simulink model "gm_wlanhdlTimeAndFrequencySynchronization"  (R2025a)
settings: Solver=FixedStepDiscrete  StartTime=0.0  StopTime=stopTime  RelTol=1e-3
InitFcn:
  | wlanFrontEndInit;
undefined symbols (not defined in the file or in its folder): a, b, c, Hd, wlanConfig
libraries: simulink x95, hdlsllib x16, hdlmdlgenlib x12, dspsrcs4 x3, dspsigops x3, dsphdlsigops2 x2, dsphdlfiltering2 x2
(part 7 of 11)

== system gm_wlanhdlTimeAndFrequencySynchronization/WLANTimeAndFrequencySynchronization/Coarse CFO Estimation and Correction/Coarse CFO Estimation/Iteration8 ==
  xin : Inport  OutDataTypeStr=fixdt(1, 32, 19)  SampleTime=6.25e-09
  yin : Inport  Port=2  OutDataTypeStr=fixdt(1, 32, 19)  SampleTime=6.25e-09
  zin : Inport  Port=3  OutDataTypeStr=fixdt(1, 34, 33)  SampleTime=6.25e-09
  lut_value : Inport  Port=4  OutDataTypeStr=fixdt(0, 31, 33)  SampleTime=6.25e-09
  idx : Inport  Port=5  OutDataTypeStr=fixdt(0, 6, 0)  SampleTime=6.25e-09
  MuxX : Switch  Criteria=u2 ~= 0  Threshold="fi(0,0,1,0,\"hex\",\"0\")"  OutDataTypeStr=fixdt(1, 32, 19)  SampleTime=6.25e-09  SaturateOnIntegerOverflow=off  InputSameDT=off
  MuxY : Switch  Criteria=u2 ~= 0  Threshold="fi(0,0,1,0,\"hex\",\"0\")"  OutDataTypeStr=fixdt(1, 32, 19)  SampleTime=6.25e-09  SaturateOnIntegerOverflow=off  InputSameDT=off
  MuxZ : Switch  Criteria=u2 ~= 0  Threshold="fi(0,0,1,0,\"hex\",\"0\")"  OutDataTypeStr=fixdt(1, 34, 33)  SampleTime=6.25e-09  SaturateOnIntegerOverflow=off  InputSameDT=off
  XAdder : Sum  OutDataTypeStr=fixdt(1, 32, 19)  SampleTime=6.25e-09
  XSubtractor : Sum  Inputs=+-  OutDataTypeStr=fixdt(1, 32, 19)  AccumDataTypeStr=fixdt(1, 32, 19)  SampleTime=6.25e-09
  YAdder : Sum  OutDataTypeStr=fixdt(1, 32, 19)  SampleTime=6.25e-09
  YSub : Sum  Inputs=+-  OutDataTypeStr=fixdt(1, 32, 19)  AccumDataTypeStr=fixdt(1, 32, 19)  SampleTime=6.25e-09
  ZAdder : Sum  OutDataTypeStr=fixdt(1, 34, 33)  SampleTime=6.25e-09
  ZSub : Sum  Inputs=+-  OutDataTypeStr=fixdt(1, 34, 33)  AccumDataTypeStr=fixdt(1, 34, 33)  SampleTime=6.25e-09
  compare : simulink/Logic and Bit Operations/Compare To Constant  relop=<  const=double(0)  OutDataTypeStr=boolean
  dynamic_shift : ArithShift  BitShiftNumberSource=Input port  BitShiftDirection=Right
      settings: InputPortMap=u0,p1
  dynamic_shift1 : ArithShift  BitShiftNumberSource=Input port  BitShiftDirection=Right
      settings: InputPortMap=u0,p1
  rd_{0..9} (10 alike) : Delay  DelayLength=double(1)  InitialCondition=0  SampleTime=6.25e-09
  xout : Outport  OutDataTypeStr=fixdt(1, 32, 19)  SampleTime=6.25e-09
  yout : Outport  Port=2  OutDataTypeStr=fixdt(1, 32, 19)  SampleTime=6.25e-09
  zout : Outport  Port=3  OutDataTypeStr=fixdt(1, 34, 33)  SampleTime=6.25e-09
  wires:
  MuxY/1 -> yout/1
  rd_4/1 -> MuxX/3
  rd_3/1 -> MuxX/2, MuxY/2, MuxZ/2
  rd_2/1 -> MuxX/1
  rd_6/1 -> MuxY/3
  rd_5/1 -> MuxY/1
  XAdder/1 -> rd_4/1
  XSubtractor/1 -> rd_2/1
  ZAdder/1 -> rd_9/1
  MuxX/1 -> xout/1
  rd_8/1 -> MuxZ/1
  ZSub/1 -> rd_8/1
  yin/1 -> rd_1/1
  xin/1 -> rd_0/1
  idx/1 -> dynamic_shift1/2, dynamic_shift/2
  rd_1/1 -> compare/1, YAdder/1, dynamic_shift1/1, YSub/1
  zin/1 -> rd_7/1
  YSub/1 -> rd_6/1
  rd_0/1 -> dynamic_shift/1, XSubtractor/1, XAdder/1
  MuxZ/1 -> zout/1
  dynamic_shift/1 -> YSub/2, YAdder/2
  YAdder/1 -> rd_5/1
  rd_9/1 -> MuxZ/3
  rd_7/1 -> ZSub/1, ZAdder/1
  compare/1 -> rd_3/1
  lut_value/1 -> ZAdder/2, ZSub/2
  dynamic_shift1/1 -> XAdder/2, XSubtractor/2

== system gm_wlanhdlTimeAndFrequencySynchronization/WLANTimeAndFrequencySynchronization/Coarse CFO Estimation and Correction/Coarse CFO Estimation/Iteration9 ==
  xin : Inport  OutDataTypeStr=fixdt(1, 32, 19)  SampleTime=6.25e-09
  yin : Inport  Port=2  OutDataTypeStr=fixdt(1, 32, 19)  SampleTime=6.25e-09
  zin : Inport  Port=3  OutDataTypeStr=fixdt(1, 34, 33)  SampleTime=6.25e-09
  lut_value : Inport  Port=4  OutDataTypeStr=fixdt(0, 31, 33)  SampleTime=6.25e-09
  idx : Inport  Port=5  OutDataTypeStr=fixdt(0, 6, 0)  SampleTime=6.25e-09
  MuxX : Switch  Criteria=u2 ~= 0  Threshold="fi(0,0,1,0,\"hex\",\"0\")"  OutDataTypeStr=fixdt(1, 32, 19)  SampleTime=6.25e-09  SaturateOnIntegerOverflow=off  InputSameDT=off
  MuxY : Switch  Criteria=u2 ~= 0  Threshold="fi(0,0,1,0,\"hex\",\"0\")"  OutDataTypeStr=fixdt(1, 32, 19)  SampleTime=6.25e-09  SaturateOnIntegerOverflow=off  InputSameDT=off
  MuxZ : Switch  Criteria=u2 ~= 0  Threshold="fi(0,0,1,0,\"hex\",\"0\")"  OutDataTypeStr=fixdt(1, 34, 33)  SampleTime=6.25e-09  SaturateOnIntegerOverflow=off  InputSameDT=off
  XAdder : Sum  OutDataTypeStr=fixdt(1, 32, 19)  SampleTime=6.25e-09
  XSubtractor : Sum  Inputs=+-  OutDataTypeStr=fixdt(1, 32, 19)  AccumDataTypeStr=fixdt(1, 32, 19)  SampleTime=6.25e-09
  YAdder : Sum  OutDataTypeStr=fixdt(1, 32, 19)  SampleTime=6.25e-09
  YSub : Sum  Inputs=+-  OutDataTypeStr=fixdt(1, 32, 19)  AccumDataTypeStr=fixdt(1, 32, 19)  SampleTime=6.25e-09
  ZAdder : Sum  OutDataTypeStr=fixdt(1, 34, 33)  SampleTime=6.25e-09
  ZSub : Sum  Inputs=+-  OutDataTypeStr=fixdt(1, 34, 33)  AccumDataTypeStr=fixdt(1, 34, 33)  SampleTime=6.25e-09
  compare : simulink/Logic and Bit Operations/Compare To Constant  relop=<  const=double(0)  OutDataTypeStr=boolean
  dynamic_shift : ArithShift  BitShiftNumberSource=Input port  BitShiftDirection=Right
      settings: InputPortMap=u0,p1
  dynamic_shift1 : ArithShift  BitShiftNumberSource=Input port  BitShiftDirection=Right
      settings: InputPortMap=u0,p1
  rd_{0..9} (10 alike) : Delay  DelayLength=double(1)  InitialCondition=0  SampleTime=6.25e-09
  xout : Outport  OutDataTypeStr=fixdt(1, 32, 19)  SampleTime=6.25e-09
  yout : Outport  Port=2  OutDataTypeStr=fixdt(1, 32, 19)  SampleTime=6.25e-09
  zout : Outport  Port=3  OutDataTypeStr=fixdt(1, 34, 33)  SampleTime=6.25e-09
  wires:
  MuxZ/1 -> zout/1
  rd_4/1 -> MuxX/3
  rd_2/1 -> MuxX/1
  MuxY/1 -> yout/1
  XAdder/1 -> rd_4/1
  XSubtractor/1 -> rd_2/1
  YAdder/1 -> rd_5/1
  yin/1 -> rd_1/1
  YSub/1 -> rd_6/1
  lut_value/1 -> ZSub/2, ZAdder/2
  rd_3/1 -> MuxX/2, MuxZ/2, MuxY/2
  compare/1 -> rd_3/1
  dynamic_shift/1 -> YAdder/2, YSub/2
  rd_5/1 -> MuxY/1
  xin/1 -> rd_0/1
  MuxX/1 -> xout/1
  zin/1 -> rd_7/1
  rd_6/1 -> MuxY/3
  rd_0/1 -> dynamic_shift/1, XSubtractor/1, XAdder/1
  idx/1 -> dynamic_shift/2, dynamic_shift1/2
  rd_8/1 -> MuxZ/1
  rd_7/1 -> ZSub/1, ZAdder/1
  rd_9/1 -> MuxZ/3
  dynamic_shift1/1 -> XSubtractor/2, XAdder/2
  ZSub/1 -> rd_8/1
  rd_1/1 -> compare/1, dynamic_shift1/1, YAdder/1, YSub/1
  ZAdder/1 -> rd_9/1

== system gm_wlanhdlTimeAndFrequencySynchronization/WLANTimeAndFrequencySynchronization/Coarse CFO Estimation and Correction/Coarse CFO Estimation/QuadrantCorrection ==
  zin : Inport  OutDataTypeStr=fixdt(1, 34, 33)  SampleTime=6.25e-09
  QA_Control : Inport  Port=2  OutDataTypeStr=fixdt(0, 5, 0)  SampleTime=6.25e-09
  Negation : Gain  Gain="fi(0,1,2,0,\"hex\",\"3\")"  ParamDataTypeStr=fixdt(1, 2, 0)  OutDataTypeStr=fixdt(1, 34, 33)  SampleTime=6.25e-09
  adder : Sum  OutDataTypeStr=fixdt(1, 34, 33)  SampleTime=6.25e-09
  dtc : hdlmdlgenlib/Buffer
  extract : simulink/Logic and Bit Operations/Extract Bits  bitsToExtract=Range of bits  numBits=8  bitIdxRange=[2 2]  outScalingMode=Treat bit field as an integer
  extract1 : simulink/Logic and Bit Operations/Extract Bits  bitsToExtract=Range of bits  numBits=8  bitIdxRange=[0 1]  outScalingMode=Treat bit field as an integer
  mux : MultiPortSwitch  DataPortOrder=Zero-based contiguous  Inputs=2  DiagnosticForDefault=None  zeroidx=on  OutDataTypeStr=fixdt(1, 34, 33)  SampleTime=6.25e-09  SaturateOnIntegerOverflow=off  InputSameDT=off
  mux1 : MultiPortSwitch  DataPortOrder=Zero-based contiguous  Inputs=4  DiagnosticForDefault=None  zeroidx=on  OutDataTypeStr=fixdt(1, 34, 33)  SampleTime=6.25e-09  SaturateOnIntegerOverflow=off  InputSameDT=off
  mux2 : MultiPortSwitch  DataPortOrder=Zero-based contiguous  Inputs=2  DiagnosticForDefault=None  zeroidx=on  OutDataTypeStr=fixdt(1, 34, 33)  SampleTime=6.25e-09  SaturateOnIntegerOverflow=off  InputSameDT=off
  mux3 : MultiPortSwitch  DataPortOrder=Zero-based contiguous  Inputs=2  DiagnosticForDefault=None  zeroidx=on  OutDataTypeStr=fixdt(1, 34, 33)  SampleTime=6.25e-09  SaturateOnIntegerOverflow=off  InputSameDT=off
  mux6out_wire : hdlmdlgenlib/Buffer
  pidivtwoconstant : Constant  Value=0.5  OutDataTypeStr=fixdt(1, 34, 33)  SampleTime=6.25e-09
  pidivtwoconstant1 : Constant  Value=0.999999999883584678173065185546875  OutDataTypeStr=fixdt(1, 34, 33)  SampleTime=6.25e-09
  pidivtwoconstant2 : Constant  Value=-1  OutDataTypeStr=fixdt(1, 34, 33)  SampleTime=6.25e-09
  pidivtwoconstant3 : Constant  Value=0  OutDataTypeStr=fixdt(1, 34, 33)  SampleTime=6.25e-09
  pidivtwosub : Sum  Inputs=+-  OutDataTypeStr=fixdt(1, 34, 33)  AccumDataTypeStr=fixdt(1, 34, 33)  SampleTime=6.25e-09
  rd_{0,2..3,6..7} (5 alike) : Delay  DelayLength=double(1)  InitialCondition=0  SampleTime=6.25e-09
  rd_{1,4..5,8..9} (5 alike) : Delay  DelayLength=double(2)  InitialCondition=0  SampleTime=6.25e-09
  slice : hdlsllib/Logic and Bit Operations/Bit Slice  lidx=double(3)  ridx=double(3)
  slice1 : hdlsllib/Logic and Bit Operations/Bit Slice  lidx=double(4)  ridx=double(4)
  subfmux : Sum  Inputs=+-  OutDataTypeStr=fixdt(1, 34, 33)  AccumDataTypeStr=fixdt(1, 34, 33)  SampleTime=6.25e-09
  zout : Outport  OutDataTypeStr=fixdt(1, 34, 33)  SampleTime=6.25e-09
  wires:
  mux6out_wire/1 -> zout/1
  pidivtwoconstant2/1 -> adder/1
  slice1/1 -> rd_1/1
  slice/1 -> rd_4/1
  pidivtwoconstant/1 -> pidivtwosub/1
  rd_0/1 -> extract/1, slice/1, slice1/1, extract1/1
  pidivtwosub/1 -> mux/2
  rd_3/1 -> rd_6/1, Negation/1
  dtc/1 -> pidivtwosub/2, mux/3
  extract/1 -> mux/1
  QA_Control/1 -> rd_0/1
  adder/1 -> rd_9/1
  Negation/1 -> rd_7/1
  extract1/1 -> rd_5/1
  rd_2/1 -> dtc/1
  mux3/1 -> mux6out_wire/1
  pidivtwoconstant1/1 -> subfmux/1, mux2/3
  rd_6/1 -> mux1/2
  rd_5/1 -> mux1/1
  subfmux/1 -> rd_8/1
  rd_7/1 -> mux1/3
  rd_8/1 -> mux1/4
  rd_9/1 -> mux1/5
  rd_1/1 -> mux3/1
  rd_4/1 -> mux2/1
  mux1/1 -> mux2/2
  mux/1 -> rd_3/1, adder/2, subfmux/2
  zin/1 -> rd_2/1
  mux2/1 -> mux3/2
  pidivtwoconstant3/1 -> mux3/3

== system gm_wlanhdlTimeAndFrequencySynchronization/WLANTimeAndFrequencySynchronization/Coarse CFO Estimation and Correction/Coarse CFO Estimation/QuadrantMapper ==
  xin : Inport  OutDataTypeStr=fixdt(1, 32, 19)  SampleTime=5e-08
  yin : Inport  Port=2  OutDataTypeStr=fixdt(1, 32, 19)  SampleTime=5e-08
  Delayin1 : UnitDelay  InitialCondition=double(0)  SampleTime=5e-08
  Delayin11 : RateTransition  InitialCondition=double(0)  OutPortSampleTimeOpt=Multiple of input port sample time  OutPortSampleTimeMultiple=8
  Delayin2 : UnitDelay  InitialCondition=double(0)  SampleTime=5e-08
  Delayin21 : RateTransition  InitialCondition=double(0)  OutPortSampleTimeOpt=Multiple of input port sample time  OutPortSampleTimeMultiple=8
  DelayxAbs : RateTransition  InitialCondition=double(0)  OutPortSampleTimeOpt=Multiple of input port sample time  OutPortSampleTimeMultiple=8
  DelayxAbs_absorbed : Delay  DelayLength=0
  DelayyAbs : RateTransition  InitialCondition=double(0)  OutPortSampleTimeOpt=Multiple of input port sample time  OutPortSampleTimeMultiple=8
  DelayyAbs_absorbed : Delay  DelayLength=0
  abs : Abs  SampleTime=6.25e-09  OutDataTypeStr=fixdt(1, 32, 19)  SaturateOnIntegerOverflow=off
  abs1 : Abs  SampleTime=6.25e-09  OutDataTypeStr=fixdt(1, 32, 19)  SaturateOnIntegerOverflow=off
  and : Logic  AllPortsSameDT=off  OutDataTypeStr=fixdt(0, 1, 0)  SampleTime=6.25e-09
  and1 : Logic  AllPortsSameDT=off  OutDataTypeStr=fixdt(0, 1, 0)  SampleTime=6.25e-09
  compare : simulink/Logic and Bit Operations/Compare To Constant  relop=<  const=double(0)  OutDataTypeStr=boolean
  compare1 : simulink/Logic and Bit Operations/Compare To Constant  relop===  const=double(0)  OutDataTypeStr=boolean
  compare2 : simulink/Logic and Bit Operations/Compare To Constant  relop=>=  const=double(0)  OutDataTypeStr=boolean
  compare3 : simulink/Logic and Bit Operations/Compare To Constant  relop=<  const=double(0)  OutDataTypeStr=boolean
  concatQCControl : hdlsllib/Logic and Bit Operations/Bit Concat  numInputs=5
  crp_out_delay : Delay  DelayLength=double(1)  InitialCondition=0  SampleTime=6.25e-09
  crp_out_delay1 : Delay  DelayLength=double(1)  InitialCondition=0  SampleTime=6.25e-09
  dtc : hdlmdlgenlib/Buffer
  dtc1 : hdlmdlgenlib/Buffer
  in0_repeat : RateTransition  Integrity=off  Deterministic=off  OutPortSampleTimeOpt=Multiple of input port sample time  OutPortSampleTimeMultiple=1/8
  in0_repeat1 : RateTransition  Integrity=off  Deterministic=off  OutPortSampleTimeOpt=Multiple of input port sample time  OutPortSampleTimeMultiple=1/8
  in1_repeat : RateTransition  Integrity=off  Deterministic=off  OutPortSampleTimeOpt=Multiple of input port sample time  OutPortSampleTimeMultiple=1/8
  in1_repeat1 : RateTransition  Integrity=off  Deterministic=off  OutPortSampleTimeOpt=Multiple of input port sample time  OutPortSampleTimeMultiple=1/8
  in2_repeat : RateTransition  Integrity=off  Deterministic=off  OutPortSampleTimeOpt=Multiple of input port sample time  OutPortSampleTimeMultiple=1/8
  in3_repeat : RateTransition  Integrity=off  Deterministic=off  OutPortSampleTimeOpt=Multiple of input port sample time  OutPortSampleTimeMultiple=1/8
  mux : MultiPortSwitch  DataPortOrder=Zero-based contiguous  Inputs=2  DiagnosticForDefault=None  zeroidx=on  OutDataTypeStr=fixdt(1, 32, 19)  SampleTime=6.25e-09  SaturateOnIntegerOverflow=off  InputSameDT=off
  mux1 : MultiPortSwitch  DataPortOrder=Zero-based contiguous  Inputs=2  DiagnosticForDefault=None  zeroidx=on  OutDataTypeStr=fixdt(1, 32, 19)  SampleTime=6.25e-09  SaturateOnIntegerOverflow=off  InputSameDT=off
  qcControl_wire : hdlmdlgenlib/Buffer
  rd_{0..10,41} (12 alike) : Delay  DelayLength=double(1)  InitialCondition=0  SampleTime=6.25e-09
  rd_01 : Delay  DelayLength=double(1)  InitialCondition=0  SampleTime=6.25e-09
  relop : RelationalOperator  Operator=>  OutDataTypeStr=fixdt(0, 1, 0)  SampleTime=6.25e-09
  xout : Outport  OutDataTypeStr=fixdt(1, 32, 19)  SampleTime=6.25e-09
  yout : Outport  Port=2  OutDataTypeStr=fixdt(1, 32, 19)  SampleTime=6.25e-09
  QA_Control : Outport  Port=3  OutDataTypeStr=fixdt(0, 5, 0)  SampleTime=6.25e-09
  wires:
  dtc/1 -> yout/1
  qcControl_wire/1 -> QA_Control/1
  mux1/1 -> dtc1/1
  concatQCControl/1 -> qcControl_wire/1
  rd_7/1 -> concatQCControl/3, mux/1, mux1/1
  dtc1/1 -> xout/1
  and/1 -> concatQCControl/2
  and1/1 -> concatQCControl/1
  rd_8/1 -> concatQCControl/5
  rd_9/1 -> mux/2, mux1/3
  rd_4/1 -> and/2, concatQCControl/4
  rd_3/1 -> and1/2
  rd_6/1 -> relop/2, rd_10/1
  crp_out_delay/1 -> DelayyAbs/1
  rd_10/1 -> mux/3, mux1/2
  crp_out_delay1/1 -> DelayxAbs/1
  yin/1 -> in0_repeat1/1
  mux/1 -> dtc/1
  DelayyAbs_absorbed/1 -> in3_repeat/1
  abs1/1 -> crp_out_delay1/1
  compare/1 -> rd_4/1
  Delayin21/1 -> Delayin2/1
  compare2/1 -> rd_3/1
  relop/1 -> rd_7/1
  compare3/1 -> rd_8/1
  rd_2/1 -> compare/1, compare2/1
  rd_01/1 -> abs/1
  abs/1 -> crp_out_delay/1
  Delayin1/1 -> in0_repeat/1
  in1_repeat/1 -> rd_0/1
  Delayin11/1 -> Delayin1/1
  rd_41/1 -> abs1/1
  in1_repeat1/1 -> Delayin11/1, rd_41/1
  rd_5/1 -> relop/1, rd_9/1
  xin/1 -> in1_repeat1/1
  DelayxAbs/1 -> DelayxAbs_absorbed/1
  DelayyAbs/1 -> DelayyAbs_absorbed/1
  in0_repeat/1 -> rd_2/1
  DelayxAbs_absorbed/1 -> in2_repeat/1
  rd_1/1 -> and/1, and1/1
  rd_0/1 -> compare1/1, compare3/1
  in0_repeat1/1 -> rd_01/1, Delayin21/1
  in3_repeat/1 -> rd_6/1
  Delayin2/1 -> in1_repeat/1
  in2_repeat/1 -> rd_5/1
  compare1/1 -> rd_1/1

== system gm_wlanhdlTimeAndFrequencySynchronization/WLANTimeAndFrequencySynchronization/Coarse CFO Estimation and Correction/Coarse CFO Estimation/Sample FreqOff ==
  freqOffIn : Inport  OutDataTypeStr=fixdt(1, 34, 33)  PortDimensions=1  SampleTime=5e-08
  enb : Inport  Port=2  OutDataTypeStr=boolean  PortDimensions=1  SampleTime=5e-08
  rst : Inport  Port=3  OutDataTypeStr=boolean  PortDimensions=1  SampleTime=5e-08
  Sample FreqOff : MATLAB Function  TreatAsAtomicUnit=on
  freqOffOut : Outport  SampleTime=5e-08  VectorParamsAs1DForOutWhenUnconnected=off
  wires:
  Sample FreqOff/1(freqOffOut) -> freqOffOut/1
  rst/1 -> Sample FreqOff/3(rst)
  enb/1 -> Sample FreqOff/2(enb)
  freqOffIn/1 -> Sample FreqOff/1(freqOffIn)

== system gm_wlanhdlTimeAndFrequencySynchronization/WLANTimeAndFrequencySynchronization/Coarse Time Sync/Correlator/MagnitudeSquared ==
  dataIn : Inport  OutDataTypeStr=fixdt(1, 33, 26)  PortDimensions=1  SampleTime=6.25e-09
      settings: SignalType=complex
  validIn : Inport  Port=2  OutDataTypeStr=boolean  PortDimensions=1  SampleTime=6.25e-09
  Add : Sum  OutDataTypeStr=fixdt(1, 66, 52)  AccumDataTypeStr=fixdt(1, 66, 52)  SampleTime=6.25e-09
  Complex to Real-Imag : ComplexToRealImag  SampleTime=6.25e-09
  Delay{,1..3} (4 alike) : Delay  DelayLength=double(1)  InitialCondition=0  SampleTime=5e-08
  Delay{4..5,11,21,31,41,61} (7 alike) : RateTransition  InitialCondition=double(0)  OutPortSampleTimeOpt=Multiple of input port sample time  OutPortSampleTimeMultiple=8
  Delay4_absorbed : Delay  DelayLength=0
  Delay5_absorbed : Delay  DelayLength=0
  Delay6 : Delay  DelayLength=double(2)  InitialCondition=0  SampleTime=5e-08
  HwModeRegister{,1..3} (4 alike) : Delay  DelayLength=double(1)  InitialCondition=0  SampleTime=6.25e-09
  PipelineRegister : Delay  DelayLength=double(1)  InitialCondition=0  SampleTime=6.25e-09
  PipelineRegister1 : Delay  DelayLength=double(1)  InitialCondition=0  SampleTime=6.25e-09
  Product1 : Product  Inputs=**  OutDataTypeStr=fixdt(1, 66, 52)  SampleTime=6.25e-09
  Product4 : Product  Inputs=**  OutDataTypeStr=fixdt(1, 66, 52)  SampleTime=6.25e-09
  crp_out_delay{,1..4} (5 alike) : Delay  DelayLength=double(1)  InitialCondition=0  SampleTime=6.25e-09
  in0_repeat : RateTransition  Integrity=off  Deterministic=off  OutPortSampleTimeOpt=Multiple of input port sample time  OutPortSampleTimeMultiple=1/8
  in1_repeat : RateTransition  Integrity=off  Deterministic=off  OutPortSampleTimeOpt=Multiple of input port sample time  OutPortSampleTimeMultiple=1/8
  in1_repeat1 : RateTransition  Integrity=off  Deterministic=off  OutPortSampleTimeOpt=Multiple of input port sample time  OutPortSampleTimeMultiple=1/8
  in2_repeat : RateTransition  Integrity=off  Deterministic=off  OutPortSampleTimeOpt=Multiple of input port sample time  OutPortSampleTimeMultiple=1/8
  in2_repeat1 : RateTransition  Integrity=off  Deterministic=off  OutPortSampleTimeOpt=Multiple of input port sample time  OutPortSampleTimeMultiple=1/8
  in3_repeat : RateTransition  Integrity=off  Deterministic=off  OutPortSampleTimeOpt=Multiple of input port sample time  OutPortSampleTimeMultiple=1/8
  rd_{0..4,11} (6 alike) : Delay  DelayLength=double(1)  InitialCondition=0  SampleTime=6.25e-09
  dataOut : Outport  SampleTime=6.25e-09  VectorParamsAs1DForOutWhenUnconnected=off
  validOut : Outport  Port=2  SampleTime=5e-08  VectorParamsAs1DForOutWhenUnconnected=off
  wires:
  rd_2/1 -> Add/2
  in1_repeat/1 -> rd_1/1
  Delay5_absorbed/1 -> in2_repeat/1
  Delay41/1 -> Delay4_absorbed/1
  crp_out_delay1/1 -> Delay41/1
  PipelineRegister1/1 -> crp_out_delay2/1
  rd_1/1 -> Add/1
  Product1/1 -> PipelineRegister1/1
  Product4/1 -> PipelineRegister/1
  crp_out_delay/1 -> Delay61/1
  rd_4/1 -> HwModeRegister3/1
  Delay21/1 -> Delay2/1
  validIn/1 -> crp_out_delay/1
  crp_out_delay3/1 -> Delay4/1, Delay11/1
  Delay1/1 -> in0_repeat/1
  Delay31/1 -> Delay3/1
  Delay/1 -> in1_repeat1/1
  Delay61/1 -> Delay6/1
  Add/1 -> dataOut/1
  in2_repeat/1 -> rd_2/1
  dataIn/1 -> Complex to Real-Imag/1
  Delay5/1 -> Delay5_absorbed/1
  PipelineRegister/1 -> crp_out_delay1/1
  Complex to Real-Imag/2 -> crp_out_delay4/1
  crp_out_delay2/1 -> Delay5/1
  Complex to Real-Imag/1 -> crp_out_delay3/1
  in0_repeat/1 -> rd_0/1
  rd_3/1 -> HwModeRegister2/1
  Delay4/1 -> Delay/1
  HwModeRegister1/1 -> Product4/2
  rd_0/1 -> HwModeRegister/1
  Delay4_absorbed/1 -> in1_repeat/1
  in1_repeat1/1 -> rd_11/1
  Delay2/1 -> in2_repeat1/1
  in2_repeat1/1 -> rd_3/1
  in3_repeat/1 -> rd_4/1
  rd_11/1 -> HwModeRegister1/1
  crp_out_delay4/1 -> Delay21/1, Delay31/1
  HwModeRegister/1 -> Product4/1
  Delay11/1 -> Delay1/1
  Delay6/1 -> validOut/1
  Delay3/1 -> in3_repeat/1
  HwModeRegister2/1 -> Product1/1
  HwModeRegister3/1 -> Product1/2

== system gm_wlanhdlTimeAndFrequencySynchronization/WLANTimeAndFrequencySynchronization/Coarse Time Sync/Correlator/MovingSum ==
  dataIn : Inport  OutDataTypeStr=fixdt(1, 32, 26)  PortDimensions=1  SampleTime=5e-08
      settings: SignalType=complex
  validIn : Inport  Port=2  OutDataTypeStr=boolean  PortDimensions=1  SampleTime=5e-08
  reset : Inport  Port=3  OutDataTypeStr=boolean  PortDimensions=1  SampleTime=5e-08
  Add : Sum  Inputs=+-  OutDataTypeStr=fixdt(1, 33, 26)  AccumDataTypeStr=fixdt(1, 33, 26)  SampleTime=6.25e-09
  Add1 : Sum  OutDataTypeStr=fixdt(1, 33, 26)  AccumDataTypeStr=fixdt(1, 33, 26)  SampleTime=6.25e-09
  Delay12 : RateTransition  InitialCondition=double(0)  OutPortSampleTimeOpt=Multiple of input port sample time  OutPortSampleTimeMultiple=8
  Delay12_absorbed : Delay  DelayLength=0
  Delay{3..6} (4 alike) : Delay  DelayLength=double(1)  InitialCondition=0  SampleTime=5e-08
  Delay31 : RateTransition  InitialCondition=double(0)  OutPortSampleTimeOpt=Multiple of input port sample time  OutPortSampleTimeMultiple=8
  Delay41 : RateTransition  InitialCondition=double(0)  OutPortSampleTimeOpt=Multiple of input port sample time  OutPortSampleTimeMultiple=8
  Delay_Switch : Switch  Criteria=u2 ~= 0  Threshold=double(0)  OutDataTypeStr=fixdt(1, 33, 26)  SampleTime=6.25e-09  SaturateOnIntegerOverflow=off  InputSameDT=off
  Shift Arithmetic : ArithShift  BitShiftNumber=double(1)  BinPtShiftNumber=double(0)
  "Synchronous Enabled 128 Sample Delay " : Subsystem
  Synchronous Enabled Unit Delay_lowered : RateTransition  InitialCondition=double(0)  OutPortSampleTimeOpt=Multiple of input port sample time  OutPortSampleTimeMultiple=8
  Synchronous Enabled Unit Delay_lowered_absorbed : Delay  DelayLength=0
  crp_out_delay : Delay  DelayLength=double(1)  InitialCondition=0  SampleTime=6.25e-09
  crp_out_delay1 : Delay  DelayLength=double(1)  InitialCondition=0  SampleTime=6.25e-09
  in0_repeat : RateTransition  Integrity=off  Deterministic=off  OutPortSampleTimeOpt=Multiple of input port sample time  OutPortSampleTimeMultiple=1/8
  in0_repeat1 : RateTransition  Integrity=off  Deterministic=off  OutPortSampleTimeOpt=Multiple of input port sample time  OutPortSampleTimeMultiple=1/8
  in1_repeat : RateTransition  Integrity=off  Deterministic=off  OutPortSampleTimeOpt=Multiple of input port sample time  OutPortSampleTimeMultiple=1/8
  in1_repeat1 : RateTransition  Integrity=off  Deterministic=off  OutPortSampleTimeOpt=Multiple of input port sample time  OutPortSampleTimeMultiple=1/8
  in2_repeat : RateTransition  Integrity=off  Deterministic=off  OutPortSampleTimeOpt=Multiple of input port sample time  OutPortSampleTimeMultiple=1/8
  in2_repeat1 : RateTransition  Integrity=off  Deterministic=off  OutPortSampleTimeOpt=Multiple of input port sample time  OutPortSampleTimeMultiple=1/8
  rd_{1..3,5,11,21,31} (7 alike) : Delay  DelayLength=double(1)  InitialCondition=0  SampleTime=6.25e-09
  rd_4 : Delay  DelayLength=double(2)  InitialCondition=0  SampleTime=6.25e-09
  dataOut : Outport  SampleTime=5e-08  VectorParamsAs1DForOutWhenUnconnected=off
  validOut : Outport  Port=2  SampleTime=5e-08  VectorParamsAs1DForOutWhenUnconnected=off
  wires:
  rd_11/1 -> Add1/1, rd_5/1
  rd_1/1 -> Add/1
  in2_repeat/1 -> rd_2/1
  rd_21/1 -> Add1/2
  in1_repeat/1 -> rd_1/1
  in1_repeat1/1 -> rd_11/1
  Delay31/1 -> Delay3/1
  reset/1 -> "Synchronous Enabled 128 Sample Delay "/3(reset)
  rd_5/1 -> Delay_Switch/3
  Delay41/1 -> Delay4/1
  crp_out_delay1/1 -> Synchronous Enabled Unit Delay_lowered/1
  Delay3/1 -> in0_repeat1/1
  rd_2/1 -> Add/2
  in0_repeat/1 -> Delay31/1
  validIn/1 -> in0_repeat/1, "Synchronous Enabled 128 Sample Delay "/2(en)
  Synchronous Enabled Unit Delay_lowered/1 -> Synchronous Enabled Unit Delay_lowered_absorbed/1
  dataIn/1 -> "Synchronous Enabled 128 Sample Delay "/1(dataIn), in1_repeat/1
  rd_4/1 -> Delay_Switch/2
  rd_31/1 -> Delay_Switch/1
  in0_repeat1/1 -> Delay41/1, rd_4/1
  rd_3/1 -> Shift Arithmetic/1
  Add1/1 -> rd_31/1
  Synchronous Enabled Unit Delay_lowered_absorbed/1 -> in1_repeat1/1, Delay5/1
  in2_repeat1/1 -> rd_21/1
  Delay12_absorbed/1 -> in2_repeat1/1
  "Synchronous Enabled 128 Sample Delay "/1(dataOut) -> in2_repeat/1
  Delay_Switch/1 -> crp_out_delay1/1
  Add/1 -> rd_3/1
  Delay4/1 -> Delay6/1
  Shift Arithmetic/1 -> crp_out_delay/1
  crp_out_delay/1 -> Delay12/1
  Delay12/1 -> Delay12_absorbed/1
  Delay6/1 -> validOut/1
  Delay5/1 -> dataOut/1

== system gm_wlanhdlTimeAndFrequencySynchronization/WLANTimeAndFrequencySynchronization/Coarse Time Sync/Correlator/delayedCorrelation ==
  dataIn : Inport  OutDataTypeStr=fixdt(1, 16, 12)  PortDimensions=1  SampleTime=5e-08
      settings: SignalType=complex
  validIn : Inport  Port=2  OutDataTypeStr=boolean  PortDimensions=1  SampleTime=5e-08
  startIn : Inport  Port=3  OutDataTypeStr=boolean  PortDimensions=1  SampleTime=5e-08
  Conjugate : Math  Operator=conj  SignedPower=on  OutDataTypeStr=fixdt(1, 16, 12)  RndMeth=Zero
  DTadjust : Subsystem
  Delay1 : Delay  DelayLength=double(16)  InitialCondition=0  SampleTime=5e-08
  Delay16 : Delay  DelayLength=double(14)  InitialCondition=0  SampleTime=5e-08
  Delay4 : Delay  DelayLength=double(2)  InitialCondition=0  SampleTime=5e-08
  Delay5 : Delay  DelayLength=double(2)  InitialCondition=0  SampleTime=5e-08
  Delay6 : RateTransition  InitialCondition=double(0)  OutPortSampleTimeOpt=Multiple of input port sample time  OutPortSampleTimeMultiple=8
  Delay6_absorbed : Delay  DelayLength=0
  Delay7 : Delay  DelayLength=double(3)  InitialCondition=0  SampleTime=5e-08
  Delay8 : Delay  DelayLength=double(3)  InitialCondition=0  SampleTime=5e-08
  HwModeRegister{,1..9} (10 alike) : Delay  DelayLength=double(1)  InitialCondition=0  SampleTime=6.25e-09
  MultiplyAdd : hdlsllib/HDL Operations/Multiply-Add  Function=c-(a.*b)  datatype=fixdt(1, 33, 24)  DoSatur=off  FMA=off
  MultiplyAdd1 : hdlsllib/HDL Operations/Multiply-Add  Function=c+(a.*b)  datatype=fixdt(1, 33, 24)  DoSatur=off  FMA=off
  MultiplyAdd_out_dtc : DataTypeConversion  OutDataTypeStr=fixdt(1, 32, 24)  SampleTime=6.25e-09  SaturateOnIntegerOverflow=off  RndMeth=Floor
  MultiplyAdd_out_dtc1 : DataTypeConversion  OutDataTypeStr=fixdt(1, 32, 24)  SampleTime=6.25e-09  SaturateOnIntegerOverflow=off  RndMeth=Floor
  PipelineRegister : Delay  DelayLength=double(1)  InitialCondition=0  SampleTime=6.25e-09
  PipelineRegister1 : Delay  DelayLength=double(1)  InitialCondition=0  SampleTime=6.25e-09
  PipelineRegister2 : Delay  DelayLength=double(2)  InitialCondition=0  SampleTime=6.25e-09
  PipelineRegister3 : Delay  DelayLength=double(2)  InitialCondition=0  SampleTime=6.25e-09
  Product : Product  Inputs=**  OutDataTypeStr=fixdt(1, 32, 24)  SampleTime=6.25e-09
  Product1 : Product  Inputs=**  OutDataTypeStr=fixdt(1, 32, 24)  SampleTime=6.25e-09
  Product_C2ReIm_1 : ComplexToRealImag  SampleTime=6.25e-09
  Product_C2ReIm_2 : ComplexToRealImag  SampleTime=6.25e-09
  Product_ReIm2Complex : RealImagToComplex  SampleTime=6.25e-09
  crp_out_delay : Delay  DelayLength=double(1)  InitialCondition=0  SampleTime=6.25e-09
  in0_repeat : RateTransition  Integrity=off  Deterministic=off  OutPortSampleTimeOpt=Multiple of input port sample time  OutPortSampleTimeMultiple=1/8
  in1_repeat : RateTransition  Integrity=off  Deterministic=off  OutPortSampleTimeOpt=Multiple of input port sample time  OutPortSampleTimeMultiple=1/8
  rd_0 : Delay  DelayLength=double(1)  InitialCondition=0  SampleTime=6.25e-09
  rd_1 : Delay  DelayLength=double(2)  InitialCondition=0  SampleTime=6.25e-09
  rd_2 : Delay  DelayLength=double(1)  InitialCondition=0  SampleTime=6.25e-09
  rd_3 : Delay  DelayLength=double(2)  InitialCondition=0  SampleTime=6.25e-09
  rd_4 : Delay  DelayLength=double(2)  InitialCondition=0  SampleTime=6.25e-09
  corrOut : Outport  SampleTime=5e-08
  corrValid : Outport  Port=2  SampleTime=5e-08
  startOut : Outport  Port=3  SampleTime=5e-08
  wires:
  Delay6_absorbed/1 -> DTadjust/1(in)
  MultiplyAdd_out_dtc1/1 -> Product_ReIm2Complex/2
  MultiplyAdd_out_dtc/1 -> Product_ReIm2Complex/1
  MultiplyAdd/1 -> PipelineRegister2/1
  HwModeRegister6/1 -> MultiplyAdd/3
  HwModeRegister4/1 -> MultiplyAdd/1
  DTadjust/1(out) -> corrOut/1
  PipelineRegister1/1 -> HwModeRegister9/1
  HwModeRegister8/1 -> MultiplyAdd1/2
  rd_0/1 -> Product_C2ReIm_1/1
  Product_ReIm2Complex/1 -> crp_out_delay/1
  rd_4/1 -> HwModeRegister8/1
  Delay5/1 -> in1_repeat/1
  Delay4/1 -> Delay16/1, in0_repeat/1
  crp_out_delay/1 -> Delay6/1
  rd_3/1 -> HwModeRegister5/1
  HwModeRegister/1 -> Product/1
  Conjugate/1 -> Delay5/1
  validIn/1 -> Delay1/1
  HwModeRegister3/1 -> Product1/2
  PipelineRegister3/1 -> MultiplyAdd_out_dtc1/1
  MultiplyAdd1/1 -> PipelineRegister3/1
  in1_repeat/1 -> rd_2/1
  dataIn/1 -> Delay4/1
  in0_repeat/1 -> rd_0/1
  Delay16/1 -> Conjugate/1
  Delay8/1 -> startOut/1
  Product1/1 -> PipelineRegister1/1
  rd_1/1 -> HwModeRegister7/1, HwModeRegister4/1
  PipelineRegister/1 -> HwModeRegister6/1
  Delay1/1 -> Delay7/1
  PipelineRegister2/1 -> MultiplyAdd_out_dtc/1
  startIn/1 -> Delay8/1
  HwModeRegister7/1 -> MultiplyAdd1/1
  Delay7/1 -> corrValid/1
  Delay6/1 -> Delay6_absorbed/1
  rd_2/1 -> Product_C2ReIm_2/1
  Product_C2ReIm_1/1 -> HwModeRegister2/1, HwModeRegister/1
  Product_C2ReIm_1/2 -> rd_1/1
  Product_C2ReIm_2/1 -> HwModeRegister1/1, rd_4/1
  HwModeRegister5/1 -> MultiplyAdd/2
  Product_C2ReIm_2/2 -> HwModeRegister3/1, rd_3/1
  HwModeRegister1/1 -> Product/2
  HwModeRegister9/1 -> MultiplyAdd1/3
  HwModeRegister2/1 -> Product1/1
  Product/1 -> PipelineRegister/1

== system gm_wlanhdlTimeAndFrequencySynchronization/WLANTimeAndFrequencySynchronization/Coarse Time Sync/Energy Calculator/magnitudeSquared ==
  dataIn : Inport  OutDataTypeStr=fixdt(1, 16, 12)  PortDimensions=1  SampleTime=5e-08
      settings: SignalType=complex
  validIn : Inport  Port=2  OutDataTypeStr=boolean  PortDimensions=1  SampleTime=5e-08
  Add : Sum  OutDataTypeStr=fixdt(1, 34, 27)  AccumDataTypeStr=fixdt(1, 34, 27)  SampleTime=6.25e-09
  Delay : Delay  DelayLength=double(16)  InitialCondition=0  SampleTime=5e-08
  Delay1 : Delay  DelayLength=double(16)  InitialCondition=0  SampleTime=5e-08
  Delay11 : RateTransition  InitialCondition=double(0)  OutPortSampleTimeOpt=Multiple of input port sample time  OutPortSampleTimeMultiple=8
  Delay2 : Delay  DelayLength=double(15)  InitialCondition=0  SampleTime=5e-08
  Delay21 : RateTransition  InitialCondition=double(0)  OutPortSampleTimeOpt=Multiple of input port sample time  OutPortSampleTimeMultiple=8
  Delay3 : RateTransition  InitialCondition=double(0)  OutPortSampleTimeOpt=Multiple of input port sample time  OutPortSampleTimeMultiple=8
  Delay3_absorbed : Delay  DelayLength=0
  Delay4 : Delay  DelayLength=double(1)  InitialCondition=0  SampleTime=5e-08
  MagnitudeSquared : Subsystem
  MagnitudeSquared1 : Subsystem
  MovingSum : Subsystem
  Shift Arithmetic : ArithShift  BitShiftNumber=double(1)  BinPtShiftNumber=double(0)
  Shift Arithmetic1 : ArithShift  BitShiftNumber=double(4)  BinPtShiftNumber=double(0)
  Shift Arithmetic2 : ArithShift  BitShiftNumber=double(1)  BinPtShiftNumber=double(0)
  crp_out_delay : Delay  DelayLength=double(1)  InitialCondition=0  SampleTime=6.25e-09
  in0_repeat : RateTransition  Integrity=off  Deterministic=off  OutPortSampleTimeOpt=Multiple of input port sample time  OutPortSampleTimeMultiple=1/8
  in0_repeat1 : RateTransition  Integrity=off  Deterministic=off  OutPortSampleTimeOpt=Multiple of input port sample time  OutPortSampleTimeMultiple=1/8
  in1_repeat : RateTransition  Integrity=off  Deterministic=off  OutPortSampleTimeOpt=Multiple of input port sample time  OutPortSampleTimeMultiple=1/8
  in1_repeat1 : RateTransition  Integrity=off  Deterministic=off  OutPortSampleTimeOpt=Multiple of input port sample time  OutPortSampleTimeMultiple=1/8
  in2_repeat : RateTransition  Integrity=off  Deterministic=off  OutPortSampleTimeOpt=Multiple of input port sample time  OutPortSampleTimeMultiple=1/8
  rd_{0..3,11} (5 alike) : Delay  DelayLength=double(1)  InitialCondition=0  SampleTime=6.25e-09
  energy : Outport  SampleTime=6.25e-09
  push : Outport  Port=2  SampleTime=5e-08
  wires:
  Delay/1 -> in2_repeat/1
  rd_1/1 -> Add/1
  Delay3_absorbed/1 -> Delay/1, in1_repeat/1
  Delay11/1 -> Delay1/1
  Shift Arithmetic2/1 -> energy/1
  in0_repeat/1 -> Delay11/1
  rd_11/1 -> Shift Arithmetic1/1
  Delay3/1 -> Delay3_absorbed/1
  Delay4/1 -> in0_repeat/1
  MagnitudeSquared/2(validOut) -> Delay4/1
  rd_2/1 -> Add/2
  in0_repeat1/1 -> Delay21/1
  validIn/1 -> MagnitudeSquared/2(validIn)
  Shift Arithmetic1/1 -> MagnitudeSquared1/1(dataIn)
  in1_repeat/1 -> rd_1/1
  Delay1/1 -> MovingSum/2(validIn)
  crp_out_delay/1 -> Delay3/1
  Delay2/1 -> MagnitudeSquared1/2(validIn)
  MagnitudeSquared/1(dataOut) -> crp_out_delay/1
  rd_3/1 -> Shift Arithmetic/1
  in2_repeat/1 -> rd_2/1
  Delay21/1 -> Delay2/1
  dataIn/1 -> MagnitudeSquared/1(dataIn)
  Add/1 -> rd_3/1
  rd_0/1 -> Shift Arithmetic2/1
  Shift Arithmetic/1 -> MovingSum/1(dataIn)
  MovingSum/1(dataOut) -> in1_repeat1/1
  MovingSum/2(validOut) -> in0_repeat1/1
  in1_repeat1/1 -> rd_11/1
  MagnitudeSquared1/1(dataOut) -> rd_0/1
  MagnitudeSquared1/2(validOut) -> push/1

== system gm_wlanhdlTimeAndFrequencySynchronization/WLANTimeAndFrequencySynchronization/Coarse Time Sync/Energy Calculator/streamSynchronizer ==
  corrValid : Inport  OutDataTypeStr=boolean  PortDimensions=1  SampleTime=5e-08
  energy : Inport  Port=2  OutDataTypeStr=fixdt(1, 71, 54)  PortDimensions=1  SampleTime=6.25e-09
  dataValid : Inport  Port=3  OutDataTypeStr=boolean  PortDimensions=1  SampleTime=5e-08
  Delay1 : RateTransition  InitialCondition=double(0)  OutPortSampleTimeOpt=Multiple of input port sample time  OutPortSampleTimeMultiple=8
  Delay1_absorbed : Delay  DelayLength=0
  Delay{2..4,6} (4 alike) : Delay  DelayLength=double(1)  InitialCondition=0  SampleTime=5e-08
  Delay41 : RateTransition  InitialCondition=double(0)  OutPortSampleTimeOpt=Multiple of input port sample time  OutPortSampleTimeMultiple=8
  Delay61 : RateTransition  InitialCondition=double(0)  OutPortSampleTimeOpt=Multiple of input port sample time  OutPortSampleTimeMultiple=8
  StreamSyncronizer : Subsystem
  crp_out_delay : Delay  DelayLength=double(1)  InitialCondition=0  SampleTime=6.25e-09
  in0_repeat : RateTransition  Integrity=off  Deterministic=off  OutPortSampleTimeOpt=Multiple of input port sample time  OutPortSampleTimeMultiple=1/8
  in1_repeat : RateTransition  Integrity=off  Deterministic=off  OutPortSampleTimeOpt=Multiple of input port sample time  OutPortSampleTimeMultiple=1/8
  dataOut : Outport  SampleTime=5e-08
  validOut : Outport  Port=2  SampleTime=5e-08
  wires:
  Delay3/1 -> validOut/1
  Delay2/1 -> dataOut/1
  StreamSyncronizer/2(validOut) -> Delay3/1
  corrValid/1 -> in0_repeat/1
  in0_repeat/1 -> Delay41/1
  energy/1 -> crp_out_delay/1
  dataValid/1 -> in1_repeat/1
  crp_out_delay/1 -> Delay1/1
  Delay1_absorbed/1 -> StreamSyncronizer/2(dataIn)
  in1_repeat/1 -> Delay61/1
  Delay41/1 -> Delay4/1
  Delay1/1 -> Delay1_absorbed/1
  Delay61/1 -> Delay6/1
  Delay4/1 -> StreamSyncronizer/1(pop)
  Delay6/1 -> StreamSyncronizer/3(push)
  StreamSyncronizer/1(dataOut) -> Delay2/1

== system gm_wlanhdlTimeAndFrequencySynchronization/WLANTimeAndFrequencySynchronization/Coarse Time Sync/Peak Detector/MATLAB Function1 ==
  syncEn : Inport  OutDataTypeStr=boolean  PortDimensions=1  SampleTime=5e-08
  dataIn : Inport  Port=2  OutDataTypeStr=fixdt(1, 16, 12)  PortDimensions=1  SampleTime=5e-08
      settings: SignalType=complex
  validIn : Inport  Port=3  OutDataTypeStr=boolean  PortDimensions=1  SampleTime=5e-08
  MATLAB Function1 : MATLAB Function  TreatAsAtomicUnit=on
  dataOut : Outport  SampleTime=5e-08  VectorParamsAs1DForOutWhenUnconnected=off
  wires:
  MATLAB Function1/1(dataOut) -> dataOut/1
  validIn/1 -> MATLAB Function1/3(validIn)
  dataIn/1 -> MATLAB Function1/2(dataIn)
  syncEn/1 -> MATLAB Function1/1(syncEn)

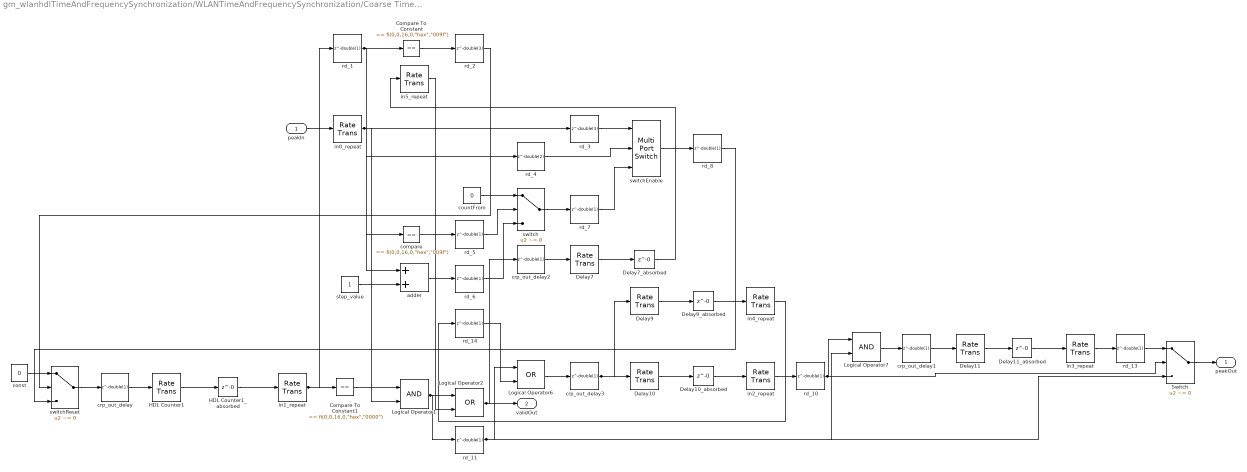
== system gm_wlanhdlTimeAndFrequencySynchronization/WLANTimeAndFrequencySynchronization/Coarse Time Sync/Peak Detector/considerFirstPeak ==
  peakIn : Inport  OutDataTypeStr=boolean  PortDimensions=1  SampleTime=5e-08
  Compare To Constant : simulink/Logic and Bit Operations/Compare To Constant  relop===  const="fi(0,0,16,0,\"hex\",\"009f\")"  OutDataTypeStr=boolean
  Compare To Constant1 : simulink/Logic and Bit Operations/Compare To Constant  relop===  const="fi(0,0,16,0,\"hex\",\"0000\")"  OutDataTypeStr=boolean
  Delay{7,9..11} (4 alike) : RateTransition  InitialCondition=double(0)  OutPortSampleTimeOpt=Multiple of input port sample time  OutPortSampleTimeMultiple=8
  Delay10_absorbed : Delay  DelayLength=0
  Delay11_absorbed : Delay  DelayLength=0
  Delay7_absorbed : Delay  DelayLength=0
  Delay9_absorbed : Delay  DelayLength=0
  HDL Counter1 : RateTransition  InitialCondition=double(0)  OutPortSampleTimeOpt=Multiple of input port sample time  OutPortSampleTimeMultiple=8
  HDL Counter1_absorbed : Delay  DelayLength=0
  Logical Operator1 : Logic  AllPortsSameDT=off  OutDataTypeStr=boolean  SampleTime=6.25e-09
  Logical Operator2 : Logic  Operator=OR  AllPortsSameDT=off  OutDataTypeStr=boolean  SampleTime=6.25e-09
  Logical Operator6 : Logic  Operator=OR  AllPortsSameDT=off  OutDataTypeStr=boolean  SampleTime=6.25e-09
  Logical Operator7 : Logic  AllPortsSameDT=off  OutDataTypeStr=boolean  SampleTime=6.25e-09
  Switch : Switch  Criteria=u2 ~= 0  Threshold="fi(0,0,1,0,\"hex\",\"0\")"  OutDataTypeStr=boolean  SampleTime=6.25e-09  SaturateOnIntegerOverflow=off  InputSameDT=off
  adder : Sum  OutDataTypeStr=uint16  AccumDataTypeStr=uint16  SampleTime=6.25e-09
  compare : simulink/Logic and Bit Operations/Compare To Constant  relop===  const="fi(0,0,16,0,\"hex\",\"009f\")"  OutDataTypeStr=boolean
  const : Constant  Value=0  VectorParams1D=off  OutDataTypeStr=uint16  SampleTime=6.25e-09
  countFrom : Constant  Value=0  VectorParams1D=off  OutDataTypeStr=uint16  SampleTime=6.25e-09
  crp_out_delay{,1..3} (4 alike) : Delay  DelayLength=double(1)  InitialCondition=0  SampleTime=6.25e-09
  in0_repeat : RateTransition  Integrity=off  Deterministic=off  OutPortSampleTimeOpt=Multiple of input port sample time  OutPortSampleTimeMultiple=1/8
  in1_repeat : RateTransition  Integrity=off  Deterministic=off  OutPortSampleTimeOpt=Multiple of input port sample time  OutPortSampleTimeMultiple=1/8
  in2_repeat : RateTransition  Integrity=off  Deterministic=off  OutPortSampleTimeOpt=Multiple of input port sample time  OutPortSampleTimeMultiple=1/8
  in3_repeat : RateTransition  Integrity=off  Deterministic=off  OutPortSampleTimeOpt=Multiple of input port sample time  OutPortSampleTimeMultiple=1/8
  in4_repeat : RateTransition  Integrity=off  Deterministic=off  OutPortSampleTimeOpt=Multiple of input port sample time  OutPortSampleTimeMultiple=1/8
  in5_repeat : RateTransition  Integrity=off  Deterministic=off  OutPortSampleTimeOpt=Multiple of input port sample time  OutPortSampleTimeMultiple=1/8
  rd_{1,5..8,10..11,13..14} (9 alike) : Delay  DelayLength=double(1)  InitialCondition=0  SampleTime=6.25e-09
  rd_2 : Delay  DelayLength=double(3)  InitialCondition=0  SampleTime=6.25e-09
  rd_3 : Delay  DelayLength=double(3)  InitialCondition=0  SampleTime=6.25e-09
  rd_4 : Delay  DelayLength=double(2)  InitialCondition=0  SampleTime=6.25e-09
  step_value : Constant  VectorParams1D=off  OutDataTypeStr=uint16  SampleTime=6.25e-09
  switch : Switch  Criteria=u2 ~= 0  Threshold="fi(0,0,1,0,\"hex\",\"0\")"  OutDataTypeStr=uint16  SampleTime=6.25e-09  SaturateOnIntegerOverflow=off  InputSameDT=off
  switchEnable : MultiPortSwitch  DataPortOrder=Zero-based contiguous  Inputs=2  DiagnosticForDefault=None  zeroidx=on  OutDataTypeStr=uint16  SampleTime=6.25e-09  SaturateOnIntegerOverflow=off  InputSameDT=off
  switchReset : Switch  Criteria=u2 ~= 0  Threshold="fi(0,0,1,0,\"hex\",\"0\")"  OutDataTypeStr=uint16  SampleTime=6.25e-09  SaturateOnIntegerOverflow=off  InputSameDT=off
  peakOut : Outport  SampleTime=6.25e-09
  validOut : Outport  Port=2  SampleTime=6.25e-09
  wires:
  Switch/1 -> peakOut/1
  rd_13/1 -> Switch/1
  in3_repeat/1 -> rd_13/1
  Delay11_absorbed/1 -> in3_repeat/1
  Delay11/1 -> Delay11_absorbed/1
  crp_out_delay1/1 -> Delay11/1
  rd_10/1 -> Logical Operator7/1, Switch/2
  in4_repeat/1 -> rd_14/1
  Delay9_absorbed/1 -> in4_repeat/1
  Delay10/1 -> Delay10_absorbed/1
  in2_repeat/1 -> rd_10/1
  Delay9/1 -> Delay9_absorbed/1
  Delay7_absorbed/1 -> in5_repeat/1
  switchEnable/1 -> rd_8/1
  crp_out_delay3/1 -> Delay10/1, Delay9/1
  Delay10_absorbed/1 -> in2_repeat/1
  Compare To Constant1/1 -> Logical Operator1/1
  adder/1 -> rd_6/1
  rd_6/1 -> switch/3
  rd_3/1 -> switchEnable/1
  HDL Counter1_absorbed/1 -> in1_repeat/1
  const/1 -> switchReset/1
  Compare To Constant/1 -> rd_2/1
  Logical Operator2/1 -> crp_out_delay2/1, validOut/1
  HDL Counter1/1 -> HDL Counter1_absorbed/1
  in5_repeat/1 -> Logical Operator2/2
  in1_repeat/1 -> rd_1/1, Compare To Constant1/1
  rd_5/1 -> switch/2
  crp_out_delay/1 -> HDL Counter1/1
  rd_1/1 -> compare/1, adder/1, Compare To Constant/1, rd_4/1
  switchReset/1 -> crp_out_delay/1
  rd_8/1 -> switchReset/3
  compare/1 -> rd_5/1
  peakIn/1 -> in0_repeat/1
  Logical Operator1/1 -> rd_11/1, Logical Operator2/1
  crp_out_delay2/1 -> Delay7/1
  Logical Operator7/1 -> crp_out_delay1/1
  rd_7/1 -> switchEnable/3
  switch/1 -> rd_7/1
  countFrom/1 -> switch/1
  rd_2/1 -> switchReset/2
  rd_4/1 -> switchEnable/2
  rd_14/1 -> Logical Operator6/2
  rd_11/1 -> Logical Operator6/1, Logical Operator7/2, Switch/3
  Delay7/1 -> Delay7_absorbed/1
  step_value/1 -> adder/2
  in0_repeat/1 -> Logical Operator1/2, rd_3/1
  Logical Operator6/1 -> crp_out_delay3/1

== system gm_wlanhdlTimeAndFrequencySynchronization/WLANTimeAndFrequencySynchronization/Coarse Time Sync/Peak Detector/searchStartOfFrame ==
  thresholdValid : Inport  OutDataTypeStr=boolean  PortDimensions=1  SampleTime=5e-08
  valid : Inport  Port=2  OutDataTypeStr=boolean  PortDimensions=1  SampleTime=5e-08
  searchStartOfFrame : MATLAB Function  TreatAsAtomicUnit=on
  syncOut : Outport  SampleTime=5e-08  VectorParamsAs1DForOutWhenUnconnected=off
  wires:
  searchStartOfFrame/1(syncOut) -> syncOut/1
  valid/1 -> searchStartOfFrame/2(valid)
  thresholdValid/1 -> searchStartOfFrame/1(thresholdValid)

== system gm_wlanhdlTimeAndFrequencySynchronization/WLANTimeAndFrequencySynchronization/Coarse Time Sync/Stream Synchronizer/StreamSyncronizer ==
  pop : Inport  OutDataTypeStr=boolean  PortDimensions=1  SampleTime=5e-08
  dataIn : Inport  Port=2  OutDataTypeStr=fixdt(1, 16, 12)  PortDimensions=1  SampleTime=5e-08
      settings: SignalType=complex
  push : Inport  Port=3  OutDataTypeStr=boolean  PortDimensions=1  SampleTime=5e-08
  StreamSyncronizer : MATLAB Function  InitFcn=Simulink.suppressDiagnostic(gcb, 'Stateflow:Runtime:DataOverflowErrorMSLD');  TreatAsAtomicUnit=on  mask{depth=256}
      mask help: Synchronize two data streams with a FIFO.
  dataOut : Outport  SampleTime=5e-08  VectorParamsAs1DForOutWhenUnconnected=off
  validOut : Outport  Port=2  SampleTime=5e-08  VectorParamsAs1DForOutWhenUnconnected=off
  wires:
  StreamSyncronizer/2(validOut) -> validOut/1
  StreamSyncronizer/1(dataOut) -> dataOut/1
  push/1 -> StreamSyncronizer/3(push)
  dataIn/1 -> StreamSyncronizer/2(dataIn)
  pop/1 -> StreamSyncronizer/1(pop)

== system gm_wlanhdlTimeAndFrequencySynchronization/WLANTimeAndFrequencySynchronization/Fine CFO Estimation and Correction/Fine CFO Correction/DTConverter ==
  dataIn1 : Inport  OutDataTypeStr=fixdt(1, 16, 12)  PortDimensions=1  SampleTime=5e-08
      settings: SignalType=complex
  dataIn2 : Inport  Port=2  OutDataTypeStr=fixdt(1, 32, 26)  PortDimensions=1  SampleTime=5e-08
      settings: SignalType=complex
  DTConverter : MATLAB Function  TreatAsAtomicUnit=on
  dataOut : Outport  SampleTime=5e-08  VectorParamsAs1DForOutWhenUnconnected=off
  wires:
  dataIn1/1 -> DTConverter/1(dataIn1)
  dataIn2/1 -> DTConverter/2(dataIn2)
  DTConverter/1(dataOut) -> dataOut/1
